simulink model "CH23_3B1"  (R2021b)
settings: Solver=ode45  StartTime=0.0  StopTime=50  RelTol=1e-3  EnableMultiTasking=on
libraries: commrandsrc2 x2, commdigbbndam3 x2, commfilt2 x2
settings Model: Creator=my2  LastModifiedBy=82102
settings SolverCC: AlgebraicLoopSolver=TrustRegion
settings DataIOCC: LimitDataPoints=on  SaveFormat=Array  SignalLoggingSaveFormat=ModelDataLogs  ReturnWorkspaceOutputs=off
settings OptimizationCC: LifeSpan=inf
settings DebuggingCC: SolverPrmCheckMsg=warning  MultiTaskDSMMsg=warning  MultiTaskCondExecSysMsg=none  FcnCallInpInsideContextMsg=warning  SFUnexpectedBacktrackingDiag=warning  SFNoUnconditionalDefaultTransitionDiag=warning  SFExecutionAtInitializationDiag=none  SFMachineParentedDataDiag=warning  ArithmeticOperatorsInVariantConditions=warning
settings HardwareCC: ProdBitPerPointer=32  ProdBitPerSizeT=32  ProdBitPerPtrDiffT=32  ProdLargestAtomicFloat=None  ProdIntDivRoundTo=Undefined  ProdEndianess=Unspecified  ProdWordSize=32  ProdHWDeviceType=32-bit Generic
settings ModelReferenceCC: PropagateSignalLabelsOutOfModel=off
settings SFSimCC: SimUseLocalCustomCode=off  CustomCodeUndefinedFunction=UseInterfaceOnly
settings RTWCC: RTWUseLocalCustomCode=off
settings CodeAppCC: StateflowObjectComments=on
settings GRTTargetCC: TargetLangStandard=C89/C90 (ANSI)  CombineOutputUpdateFcns=off  GRTInterface=on
settings ConfigComp: CovMetricSettings=dw  CovSaveCumulativeToWorkspaceVar=on  CovSaveSingleToWorkspaceVar=on  CovExternalEMLEnable=off

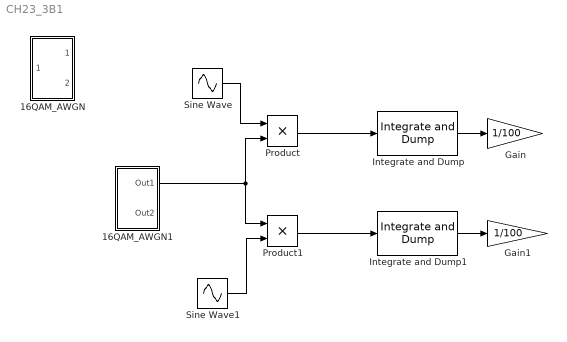
== system CH23_3B1 ==
  16QAM_AWGN : Subsystem
  16QAM_AWGN1 : Subsystem
  Gain : Gain  Gain=1/100
  Gain1 : Gain  Gain=1/100
  Integrate and Dump : commfilt2/Integrate and Dump  obssamples=100  offsetsamples=0  nodump=off  roundingMode=Floor  overflowMode=off  outputDataTypeStr=Inherit: Same as accumulator  outputLastDataTypeStr=Inherit: Same as accumulator
  Integrate and Dump1 : commfilt2/Integrate and Dump  obssamples=100  offsetsamples=0  nodump=off  roundingMode=Floor  overflowMode=off  outputDataTypeStr=Inherit: Same as accumulator  outputLastDataTypeStr=Inherit: Same as accumulator
  Product : Product
  Product1 : Product
  Sine Wave : Sin  Amplitude=sqrt(2)  Frequency=20*pi*20  Phase=pi/2  SampleTime=1/100
  Sine Wave1 : Sin  Amplitude=sqrt(2)  Frequency=2*pi*20  SampleTime=1/100
  wires:
  Sine Wave/1 -> Product/1
  16QAM_AWGN1/1(Out1) -> Product/2, Product1/1
  Sine Wave1/1 -> Product1/2
  Product/1 -> Integrate and Dump/1
  Product1/1 -> Integrate and Dump1/1
  Integrate and Dump/1 -> Gain/1
  Integrate and Dump1/1 -> Gain1/1

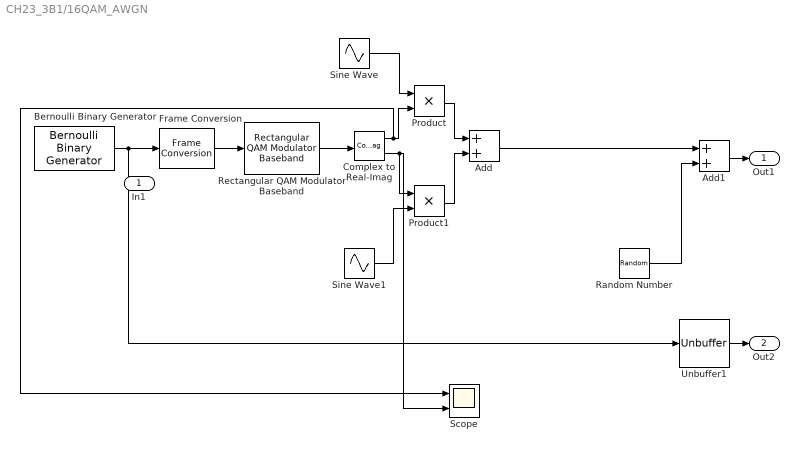
== system CH23_3B1/16QAM_AWGN ==
  In1 : Inport
  Add : Sum
  Add1 : Sum
  Bernoulli Binary Generator : commrandsrc2/Bernoulli Binary Generator  P=0.5  seed=20301181  Ts=1  frameBased=on  sampPerFrame=4  orient=off  outDataType=boolean
      settings: SourceProductBaseCode=CM
  Complex to Real-Imag : ComplexToRealImag
  Frame Conversion : FrameConversion  OutFrame=Sample-based
  Product : Product
  Product1 : Product
  Random Number : RandomNumber  Variance=0  Seed=41  SampleTime=1/100  VectorParams1D=off
  Rectangular QAM Modulator Baseband : commdigbbndam3/Rectangular QAM Modulator Baseband  M=16  InType=Bit  Enc=Gray  Mapping=[0:15]  PowType=Min. distance between symbols  MinDist=2  AvgPow=1  PeakPow=1  Ph=0  outDtype=double  outWordLen=16  outUDDataType=sfix(16)  outFracLenMode=Best precision  outFracLen=15  outDataTypeStr=double  outLastDataTypeStr=double
  Scope : Scope  NumInputPorts=2
  Sine Wave : Sin  SampleTime=1/100
  Sine Wave1 : Sin  SampleTime=1/100
  Unbuffer1 : Unbuffer
  Out1 : Outport
  Out2 : Outport  Port=2
  wires:
  Complex to Real-Imag/2 -> Scope/2, Product1/1
  Unbuffer1/1 -> Out2/1
  Add1/1 -> Out1/1
  Random Number/1 -> Add1/2
  Complex to Real-Imag/1 -> Scope/1, Product/2
  Sine Wave/1 -> Product/1
  Rectangular QAM Modulator Baseband/1 -> Complex to Real-Imag/1
  Frame Conversion/1 -> Rectangular QAM Modulator Baseband/1
  Bernoulli Binary Generator/1 -> Frame Conversion/1, Unbuffer1/1
  Product/1 -> Add/1
  Sine Wave1/1 -> Product1/2
  Add/1 -> Add1/1
  Product1/1 -> Add/2

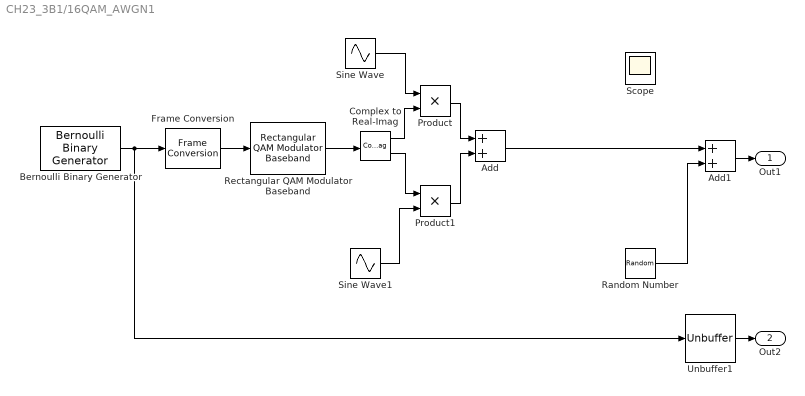
== system CH23_3B1/16QAM_AWGN1 ==
  Add : Sum
  Add1 : Sum
  Bernoulli Binary Generator : commrandsrc2/Bernoulli Binary Generator  P=0.5  seed=25  Ts=1  frameBased=on  sampPerFrame=4  orient=off  outDataType=boolean
      settings: SourceProductBaseCode=CM
  Complex to Real-Imag : ComplexToRealImag
  Frame Conversion : FrameConversion  OutFrame=Sample-based
  Product : Product
  Product1 : Product
  Random Number : RandomNumber  Variance=10  Seed=41  SampleTime=1/100  VectorParams1D=off
  Rectangular QAM Modulator Baseband : commdigbbndam3/Rectangular QAM Modulator Baseband  M=16  InType=Bit  Enc=Gray  Mapping=[0:15]  PowType=Min. distance between symbols  MinDist=2  AvgPow=1  PeakPow=1  Ph=0  outDtype=double  outWordLen=16  outUDDataType=sfix(16)  outFracLenMode=Best precision  outFracLen=15  outDataTypeStr=double  outLastDataTypeStr=double
  Scope : Scope
  Sine Wave : Sin  Amplitude=sqrt(2)  Frequency=2*pi*20  Phase=pi/2  SampleTime=1/100
  Sine Wave1 : Sin  Amplitude=sqrt(2)  Frequency=2*pi*20  SampleTime=1/100
  Unbuffer1 : Unbuffer
  Out1 : Outport
  Out2 : Outport  Port=2
  wires:
  Bernoulli Binary Generator/1 -> Frame Conversion/1, Unbuffer1/1
  Complex to Real-Imag/2 -> Product1/1
  Unbuffer1/1 -> Out2/1
  Product1/1 -> Add/2
  Random Number/1 -> Add1/2
  Add/1 -> Add1/1
  Product/1 -> Add/1
  Rectangular QAM Modulator Baseband/1 -> Complex to Real-Imag/1
  Complex to Real-Imag/1 -> Product/2
  Sine Wave1/1 -> Product1/2
  Frame Conversion/1 -> Rectangular QAM Modulator Baseband/1
  Sine Wave/1 -> Product/1
  Add1/1 -> Out1/1
